simulink model "ROV_Simulation_openloop_ver3_1"  (R2023a)
settings: Solver=ode45  StartTime=0.0  StopTime=Sim.ts  FixedStep=0.01  MaxStep=0.001  MinStep=0.00001  RelTol=1e-3
undefined symbols (not defined in the file): ext, hyd, ics, P0, P1, P10, P2, P3, P4, P5, P6, P7, P8, P9, phy, rb, thrust, VC
libraries: simulink_extras x3, simulink x1
(part 1 of 2)
settings Model: Creator=dmmavani  LastModifiedBy=dmmavani
settings SolverCC: ConcurrentTasks=on  PositivePriorityOrder=on  AutoInsertRateTranBlk=on
settings DataIOCC: InspectSignalLogs=on
settings OptimizationCC: BlockReduction=off  DefaultParameterBehavior=Inlined  EnhancedBackFolding=on  PassReuseOutputArgsAs=Individual arguments  ZeroExternalMemoryAtStartup=off  ZeroInternalMemoryAtStartup=off  OptimizeBlockOrder=speed  DifferentSizesBufferReuse=on  OptimizationCustomize=off  EfficientTunableParamExpr=on
settings DebuggingCC: TasksWithSamePriorityMsg=none  ParameterTunabilityLossMsg=error
settings HardwareCC: ProdBitPerLong=64  ProdLongLongMode=on  ProdHWDeviceType=Intel->x86-64 (Linux 64)
settings SFSimCC: MATLABDynamicMemAlloc=off
settings RTWCC: Description=Embedded Coder  SystemTargetFile=ert.tlc  GenCodeOnly=on  TemplateMakefile=ert_default_tmf  Toolchain=Simulink Real-Time Toolchain  BuildConfiguration=Faster Runs  CodeExecutionProfiling=on  TargetLang=C++
settings CodeAppCC: ForceParamTrailComments=on  IgnoreCustomStorageClasses=off  OperatorAnnotations=on  SimulinkDataObjDesc=on  SFDataObjDesc=on  InsertBlockDesc=on
settings ERTTargetCC: TargetLangStandard=C++03 (ISO)  GenerateSampleERTMain=on  CodeInterfacePackaging=C++ class  InlinedParameterPlacement=NonHierarchical  RootIOFormat=Structure reference  ERTCustomFileTemplate=example_file_process.tlc

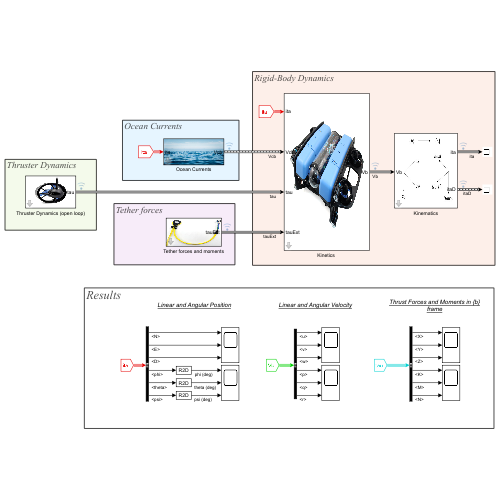
[thumbnail: Simulink's stored preview of the top-level diagram]
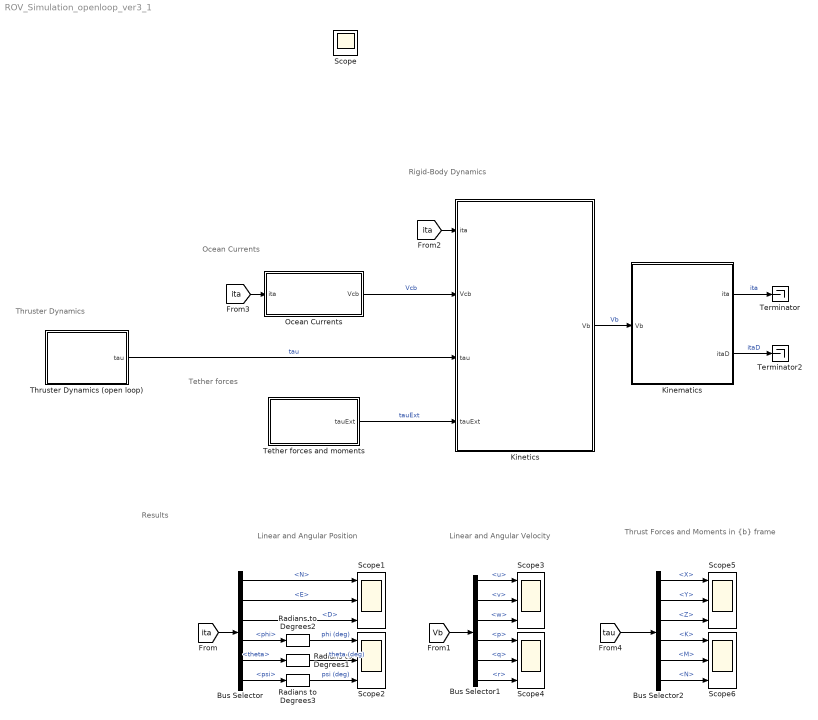
== system ROV_Simulation_openloop_ver3_1 ==
  note: Results
  note: Linear and Angular Position
  note: Tether forces
  note: Thruster Dynamics
  note: Ocean Currents
  note: Rigid-Body Dynamics
  note: Linear and Angular Velocity
  note: Thrust Forces and Moments in {b} frame
  Bus Selector : BusSelector  OutputSignals=N,E,D,phi,theta,psi
  Bus Selector1 : BusSelector  OutputSignals=u,v,w,p,q,r
  Bus Selector2 : BusSelector  OutputSignals=X,Y,Z,K,M,N
  Kinematics : Subsystem  mask{Parameter7=|, North=ics.ita.N, East=ics.ita.E, Down=ics.ita.D, Roll=ics.ita.phi, Pitch=ics.ita.theta, InitialCondition=ics.ita.psi}
      mask Parameter7=|
      | Kinematics block is used to transform velocities from BODY to
      | NED frame.
      |
      | itaD = J(euler) * Vb    ( Velocities in NED frame)
      | J(euler) = Transformation Matrix (function of euler angles)
      | Vb = Velocities in BODY frame.
      mask prompts: North "N :"; East "E :"; Down "D :"; Roll "Roll :"; Pitch "Pitch :"; InitialCondition "Yaw :"
      mask TypeOptions North: Integrator/InitialCondition
      mask TypeOptions East: Integrator1/InitialCondition
      mask TypeOptions Down: Integrator3/InitialCondition
      mask TypeOptions Roll: Integrator4/InitialCondition
      mask TypeOptions Pitch: Integrator5/InitialCondition
      mask TypeOptions InitialCondition: Integrator6/InitialCondition
      mask DialogControl Container4 Prompt: Description
      mask DialogControl Container1 Prompt: Initial Conditions for position and orientation in NED frame
      mask DialogControl Container2 Prompt: Position (meters)
      mask DialogControl Container3 Prompt: Orientation (rad)
      mask Display:
      | image('C:\Users\Dizzy\Documents\Research\MATLAB files\ROV_Simulation\documents\frame_transform_1.png.jpg');
      | port_label('input', 1, 'Vb');
      | port_label('output', 1, 'ita');
      | port_label('output', 2, 'itaD');
  "Kinetics " : Subsystem  mask{Parameter7=|, u_b=ics.vb.u, v_b=ics.vb.v, w_b=ics.vb.w, p_b=ics.vb.p, q_b=ics.vb.q, r_b=ics.vb.r}
      mask Parameter7=|
      | Kinetics block is used to solve the 6DOF equations of motion
      | of a ROV in BODY frame.
      | Block outputs V_b (Velocities in BODY frame).
      mask prompts: u_b "u :"; v_b "v :"; w_b "w :"; p_b "p :"; q_b "q :"; r_b "r :"
      mask TypeOptions u_b: Integrator/InitialCondition
      mask TypeOptions v_b: Integrator1/InitialCondition
      mask TypeOptions w_b: Integrator2/InitialCondition
      mask TypeOptions p_b: Integrator3/InitialCondition
      mask TypeOptions q_b: Integrator4/InitialCondition
      mask TypeOptions r_b: Integrator5/InitialCondition
      mask DialogControl Container4 Prompt: Description
      mask DialogControl InitialCondition Prompt: Initial conditions for velocity of body in {b} frame
      mask DialogControl Container2 Prompt: Linear Velocity  (m/s)
      mask DialogControl Container3 Prompt: Angular Velocity (rad/s)
      mask Display:
      | image('C:\Users\Dizzy\Documents\Research\MATLAB files\ROV_Simulation\documents\heavy-tutorial-21.jpg');
      | port_label('input', 1, 'ita');
      | port_label('input', 2, 'Vcb');
      | port_label('input', 3, 'tau');
      | port_label('input', 4, 'tauExt');
      | port_label('output', 1, 'Vb');
  Ocean Currents : Subsystem  mask{Parameter1=|, Value=VC}
      mask Parameter1=|
      | If the value is equal to 1 then ocean currents is ON.
      | if the value is equal to 0 then ocean currents is OFF.
      mask prompts: Value "Ocean currents (On/Off):"
      mask TypeOptions Value: Constant1/Value
      mask DialogControl Container2 Prompt: Description
      mask Display:
      | image('C:\Users\Dizzy\Documents\Research\MATLAB files\ROV_Simulation\documents\ROV_Simulation_openloop\Images\ocean_currents.jpg');
      | port_label('input', 1, 'ita');
      | port_label('output', 1, 'Vcb');
  Radians to Degrees1 : simulink_extras/Transformations/Radians to Degrees
  Radians to Degrees2 : simulink_extras/Transformations/Radians to Degrees
  Radians to Degrees3 : simulink_extras/Transformations/Radians to Degrees
  Scope{1..6} (6 alike) : Scope  NumInputPorts=3
  Terminator : Terminator
  Terminator2 : Terminator
  Tether forces and moments : Subsystem  mask(Tether forces (external forces)){}
      mask Help:
      | This block is used to compute tether forces acting on ROV in BODY or {b} frame.
      | tauExt = {Xe,Ye,Ze,Ke,Me,Ne}
      | 
      | Tether is modelled using lumped mass approach and there are certain steps to follow to alter the number of nodes for lumped mass tether model.
      | The steps are as follows:
      |     Step 1: Go inside the mask. (click on the bottom left arrow to go inside the mask)
      |     Step 2: Go inside the "tether forces" subsystem block.
      |     Step 3: Go inside the "enable" subsytem variant block.
      |     Step 4: Open MATLAB function block "Tether dynamics" and edit
      |                  the value of "n" for number of nodes.
      | 
      | ** Note **
      | The value of "n" should be two less than the total number of nodes, and must be altered everytime you change its value in workspace. Consequently, it can lead to size missmatch error if not changed.
      mask DialogControl DescGroupVar Prompt: Description
      mask DialogControl Control1 Prompt: Click on help to understand the usage of this block
      mask Display:
      | image('C:\Users\Dizzy\Documents\Research\MATLAB files\ROV_Simulation\documents\ROV_Simulation_openloop\Images\tether.jpg');
      | port_label('output', 1, 'tauExt');
  Thruster Dynamics (open loop) : Subsystem  mask{Parameter2=|, Value=1}
      mask Parameter2=|
      | Pulse input    (Input type = 1)
      | Impulse input (Input type = 0)
      mask prompts: Value "Input type:"
      mask TypeOptions Value: Constant/Value
      mask DialogControl DescGroupVar Prompt: Description
      mask Display:
      | image('C:\Users\Dizzy\Documents\Research\MATLAB files\ROV_Simulation\documents\ROV_Simulation_openloop\Images\T200-Marine-thruster.jpeg');
      | port_label('output', 1, 'tau');
  Scope : Scope
  wires:
  Ocean Currents/1(Vcb) -> "Kinetics "/2(Vcb)  "Vcb"
  [ita] -> Bus Selector/1
  Bus Selector/1 -> Scope1/1  "<N>"
  Bus Selector/2 -> Scope1/2  "<E>"
  Bus Selector/3 -> Scope1/3  "<D>"
  Bus Selector/4 -> Radians to Degrees2/1  "<phi>"
  Radians to Degrees2/1 -> Scope2/1  "phi (deg)"
  Bus Selector/5 -> Radians to Degrees1/1  "<theta>"
  Bus Selector/6 -> Radians to Degrees3/1  "<psi>"
  [Vb] -> Bus Selector1/1
  Bus Selector1/1 -> Scope3/1  "<u>"
  Bus Selector1/2 -> Scope3/2  "<v>"
  Bus Selector1/3 -> Scope3/3  "<w>"
  Bus Selector1/4 -> Scope4/1  "<p>"
  Bus Selector1/5 -> Scope4/2  "<q>"
  Bus Selector1/6 -> Scope4/3  "<r>"
  Kinematics/1(ita) -> Terminator/1  "ita"
  [ita] -> Ocean Currents/1(ita)
  Thruster Dynamics (open loop)/1(tau) -> "Kinetics "/3(tau)  "tau"
  "Kinetics "/1(Vb) -> Kinematics/1(Vb)  "Vb"
  Kinematics/2(itaD) -> Terminator2/1  "itaD"
  [ita] -> "Kinetics "/1(ita)
  [tau] -> Bus Selector2/1
  Bus Selector2/1 -> Scope5/1  "<X>"
  Bus Selector2/2 -> Scope5/2  "<Y>"
  Bus Selector2/3 -> Scope5/3  "<Z>"
  Bus Selector2/4 -> Scope6/1  "<K>"
  Bus Selector2/5 -> Scope6/2  "<M>"
  Bus Selector2/6 -> Scope6/3  "<N>"
  Radians to Degrees1/1 -> Scope2/2  "theta (deg)"
  Radians to Degrees3/1 -> Scope2/3  "psi (deg)"
  Tether forces and moments/1(tauExt) -> "Kinetics "/4(tauExt)  "tauExt"

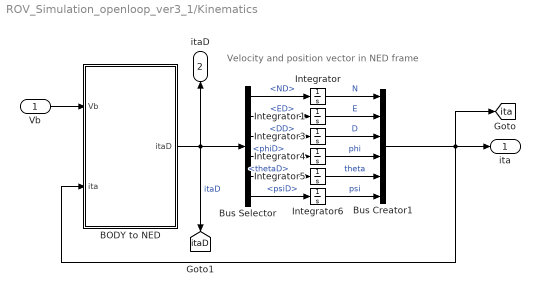
== system ROV_Simulation_openloop_ver3_1/Kinematics ==
  note: Velocity and position vector in
      |  NED frame
  Vb : Inport  OutDataTypeStr=Bus: Vb
  " BODY to NED" : MATLAB Function  TreatAsAtomicUnit=on
  Bus Creator1 : BusCreator  Inputs=6  OutDataTypeStr=Bus: ita
  Bus Selector : BusSelector  OutputSignals=ND,ED,DD,phiD,thetaD,psiD
  Integrator : Integrator  InitialCondition=North  LowerSaturationLimit=ics.N
  Integrator1 : Integrator  InitialCondition=East  LowerSaturationLimit=ics.E
  Integrator3 : Integrator  InitialCondition=Down  LowerSaturationLimit=ics.D
  Integrator4 : Integrator  InitialCondition=Roll  LowerSaturationLimit=ics.phi
  Integrator5 : Integrator  InitialCondition=Pitch  LowerSaturationLimit=ics.theta
  Integrator6 : Integrator  InitialCondition=InitialCondition  LowerSaturationLimit=ics.psi
  ita : Outport  OutDataTypeStr=Bus: ita
  itaD : Outport  Port=2  OutDataTypeStr=Bus: itaD
  tag scope: ita=global, itaD=global
  wires:
  " BODY to NED"/1(itaD) -> Bus Selector/1, [itaD], itaD/1  "itaD"
  Bus Creator1/1 -> [ita], ita/1, " BODY to NED"/2(ita)
  Bus Selector/1 -> Integrator/1  "<ND>"
  Bus Selector/2 -> Integrator1/1  "<ED>"
  Bus Selector/6 -> Integrator6/1  "<psiD>"
  Bus Selector/5 -> Integrator5/1  "<thetaD>"
  Bus Selector/3 -> Integrator3/1  "<DD>"
  Bus Selector/4 -> Integrator4/1  "<phiD>"
  Integrator/1 -> Bus Creator1/1  "N"
  Integrator1/1 -> Bus Creator1/2  "E"
  Integrator3/1 -> Bus Creator1/3  "D"
  Integrator4/1 -> Bus Creator1/4  "phi"
  Integrator5/1 -> Bus Creator1/5  "theta"
  Integrator6/1 -> Bus Creator1/6  "psi"
  Vb/1 -> " BODY to NED"/1(Vb)

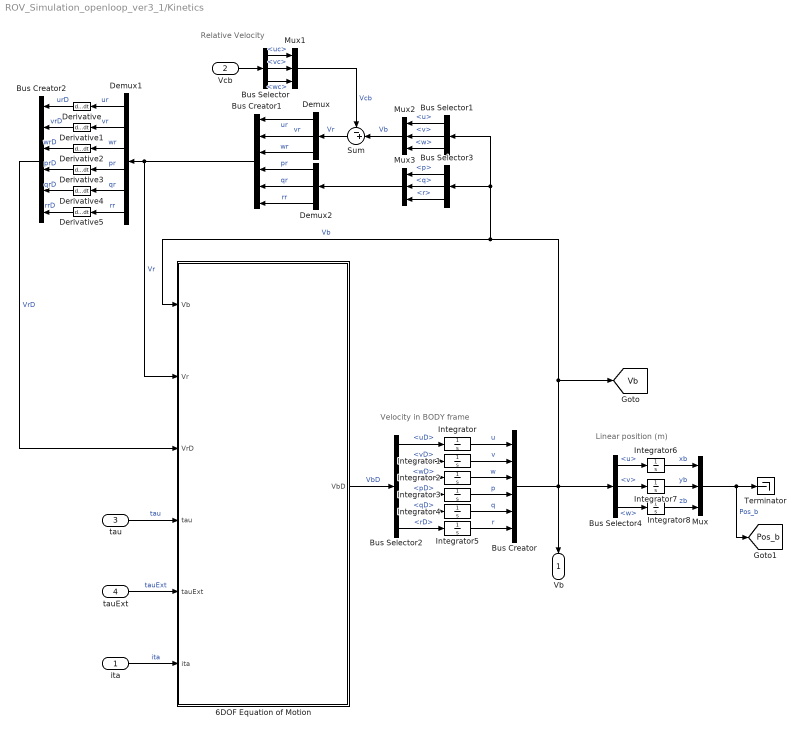
== system ROV_Simulation_openloop_ver3_1/Kinetics  ==
  note: Linear position (m)
  note: Velocity in BODY frame
  note: Relative Velocity
  ita : Inport  OutDataTypeStr=Bus: ita
  Vcb : Inport  Port=2  OutDataTypeStr=Bus: Vcb
  tau : Inport  Port=3  OutDataTypeStr=Bus: tau
  tauExt : Inport  Port=4  OutDataTypeStr=Bus: tauExt
  "6DOF Equation of Motion " : MATLAB Function  TreatAsAtomicUnit=on
  Bus Creator : BusCreator  Inputs=6  OutDataTypeStr=Bus: Vb
  Bus Creator1 : BusCreator  Inputs=6  OutDataTypeStr=Bus: Vr
  Bus Creator2 : BusCreator  Inputs=6  OutDataTypeStr=Bus: VrD
  Bus Selector : BusSelector  OutputSignals=uc,vc,wc
  Bus Selector1 : BusSelector  OutputSignals=u,v,w
  Bus Selector2 : BusSelector  OutputSignals=uD,vD,wD,pD,qD,rD
  Bus Selector3 : BusSelector  OutputSignals=p,q,r
  Bus Selector4 : BusSelector  OutputSignals=u,v,w
  Demux : Demux  Outputs=3
  Demux1 : Demux  Outputs=6
  Demux2 : Demux  Outputs=3
  Derivative{,1..5} (6 alike) : Derivative
  Integrator : Integrator  InitialCondition=u_b  UpperSaturationLimit=ics.sat.umax  LowerSaturationLimit=0
  Integrator1 : Integrator  InitialCondition=v_b  UpperSaturationLimit=ics.sat.vmax  LowerSaturationLimit=0
  Integrator2 : Integrator  InitialCondition=w_b  UpperSaturationLimit=ics.sat.wmax  LowerSaturationLimit=0
  Integrator3 : Integrator  InitialCondition=p_b  UpperSaturationLimit=ics.sat.pmax  LowerSaturationLimit=0
  Integrator4 : Integrator  InitialCondition=q_b  UpperSaturationLimit=ics.sat.qmax  LowerSaturationLimit=0
  Integrator5 : Integrator  InitialCondition=r_b  UpperSaturationLimit=ics.sat.rmax  LowerSaturationLimit=0
  Integrator6 : Integrator  LowerSaturationLimit=0
  Integrator7 : Integrator  LowerSaturationLimit=0
  Integrator8 : Integrator  LowerSaturationLimit=0
  Mux{,1..3} (4 alike) : Mux  Inputs=3
  Sum : Sum  Inputs=-+|
  Terminator : Terminator
  Vb : Outport  OutDataTypeStr=Bus: Vb
  tag scope: Pos_b=global, Vb=global
  wires:
  Mux1/1 -> Sum/1  "Vcb"
  Bus Selector1/1 -> Mux2/1  "<u>"
  Bus Selector1/2 -> Mux2/2  "<v>"
  Bus Selector1/3 -> Mux2/3  "<w>"
  Mux2/1 -> Sum/2  "Vb"
  Bus Creator/1 -> Bus Selector1/1, Bus Selector3/1, "6DOF Equation of Motion "/1(Vb), [Vb], Vb/1, Bus Selector4/1  "Vb"
  ita/1 -> "6DOF Equation of Motion "/6(ita)  "ita"
  tau/1 -> "6DOF Equation of Motion "/4(tau)  "tau"
  "6DOF Equation of Motion "/1(VbD) -> Bus Selector2/1  "VbD"
  Bus Selector2/1 -> Integrator/1  "<uD>"
  Bus Selector2/2 -> Integrator1/1  "<vD>"
  Bus Selector2/3 -> Integrator2/1  "<wD>"
  Bus Selector2/4 -> Integrator3/1  "<pD>"
  Bus Selector2/5 -> Integrator4/1  "<qD>"
  Bus Selector2/6 -> Integrator5/1  "<rD>"
  Vcb/1 -> Bus Selector/1
  Bus Selector/1 -> Mux1/1  "<uc>"
  Bus Selector/2 -> Mux1/2  "<vc>"
  Bus Selector/3 -> Mux1/3  "<wc>"
  Sum/1 -> Demux/1  "Vr"
  Demux/1 -> Bus Creator1/1  "ur"
  Demux/3 -> Bus Creator1/3  "wr"
  Mux3/1 -> Demux2/1
  Demux/2 -> Bus Creator1/2  "vr"
  Demux2/1 -> Bus Creator1/4  "pr"
  Demux2/2 -> Bus Creator1/5  "qr"
  Demux2/3 -> Bus Creator1/6  "rr"
  Integrator/1 -> Bus Creator/1  "u"
  Integrator1/1 -> Bus Creator/2  "v"
  Integrator2/1 -> Bus Creator/3  "w"
  Integrator3/1 -> Bus Creator/4  "p"
  Integrator4/1 -> Bus Creator/5  "q"
  Integrator5/1 -> Bus Creator/6  "r"
  Bus Selector3/2 -> Mux3/2  "<q>"
  Bus Selector3/3 -> Mux3/3  "<r>"
  Bus Selector3/1 -> Mux3/1  "<p>"
  Bus Selector4/1 -> Integrator6/1  "<u>"
  Bus Selector4/2 -> Integrator7/1  "<v>"
  Bus Selector4/3 -> Integrator8/1  "<w>"
  Integrator6/1 -> Mux/1  "xb"
  Integrator7/1 -> Mux/2  "yb"
  Integrator8/1 -> Mux/3  "zb"
  Mux/1 -> [Pos_b], Terminator/1  "Pos_b"
  Bus Creator1/1 -> Demux1/1, "6DOF Equation of Motion "/2(Vr)  "Vr"
  Demux1/1 -> Derivative/1  "ur"
  Derivative/1 -> Bus Creator2/1  "urD"
  Demux1/2 -> Derivative1/1  "vr"
  Derivative1/1 -> Bus Creator2/2  "vrD"
  Demux1/3 -> Derivative2/1  "wr"
  Derivative2/1 -> Bus Creator2/3  "wrD"
  Demux1/4 -> Derivative3/1  "pr"
  Derivative3/1 -> Bus Creator2/4  "prD"
  Demux1/5 -> Derivative4/1  "qr"
  Derivative4/1 -> Bus Creator2/5  "qrD"
  Demux1/6 -> Derivative5/1  "rr"
  Derivative5/1 -> Bus Creator2/6  "rrD"
  Bus Creator2/1 -> "6DOF Equation of Motion "/3(VrD)  "VrD"
  tauExt/1 -> "6DOF Equation of Motion "/5(tauExt)  "tauExt"

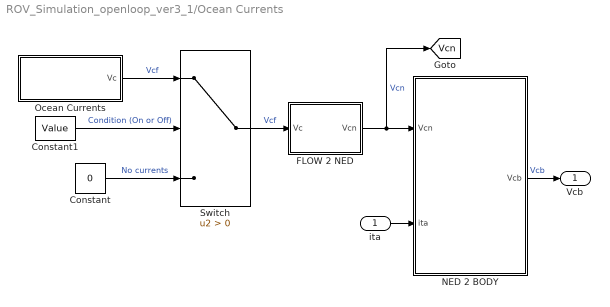
== system ROV_Simulation_openloop_ver3_1/Ocean Currents ==
  ita : Inport  OutDataTypeStr=Bus: ita
  Constant : Constant  Value=0
  Constant1 : Constant  Value=Value
  FLOW 2 NED : MATLAB Function  TreatAsAtomicUnit=on
  NED 2 BODY : MATLAB Function  TreatAsAtomicUnit=on
  Ocean Currents : Subsystem  Variant=on
  Switch : Switch  Criteria=u2 > Threshold  SaturateOnIntegerOverflow=off  InputSameDT=off
  Vcb : Outport  OutDataTypeStr=Bus: Vcb
  tag scope: Vcn=global
  wires:
  Ocean Currents/1(Vc) -> Switch/1  "Vcf"
  Constant/1 -> Switch/3  "No currents"
  Switch/1 -> FLOW 2 NED/1(Vc)  "Vcf"
  Constant1/1 -> Switch/2  "Condition (On or Off)"
  FLOW 2 NED/1(Vcn) -> NED 2 BODY/1(Vcn), [Vcn]  "Vcn"
  ita/1 -> NED 2 BODY/2(ita)
  NED 2 BODY/1(Vcb) -> Vcb/1  "Vcb"

== system ROV_Simulation_openloop_ver3_1/Tether forces and moments ==
  Tether Forces : Subsystem  Variant=on
  tauExt : Outport
  wires:
  Tether Forces/1(tauExt) -> tauExt/1

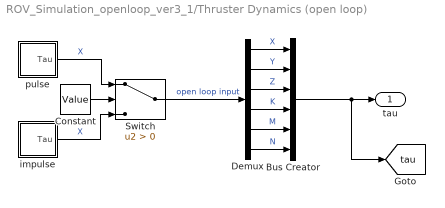
== system ROV_Simulation_openloop_ver3_1/Thruster Dynamics (open loop) ==
  Bus Creator : BusCreator  Inputs=6  OutDataTypeStr=Bus: tau
  Constant : Constant  Value=Value
  Demux : Demux  Outputs=6
  Switch : Switch  Criteria=u2 > Threshold  SaturateOnIntegerOverflow=off  InputSameDT=off
  impulse : Subsystem
  pulse : Subsystem
  tau : Outport  OutDataTypeStr=Bus: tau
  tag scope: tau=global
  wires:
  Demux/2 -> Bus Creator/2  "Y"
  Demux/3 -> Bus Creator/3  "Z"
  Demux/4 -> Bus Creator/4  "K"
  Demux/5 -> Bus Creator/5  "M"
  Demux/6 -> Bus Creator/6  "N"
  Bus Creator/1 -> [tau], tau/1
  Demux/1 -> Bus Creator/1  "X"
  pulse/1(Tau) -> Switch/1  "X"
  impulse/1(Tau) -> Switch/3  "X"
  Constant/1 -> Switch/2
  Switch/1 -> Demux/1  "open loop input"

== system ROV_Simulation_openloop_ver3_1/Ocean Currents/Ocean Currents ==
  VC_CONSTANT : Subsystem  VariantControl=VC_CONSTANT
  VC_RANDOM : Subsystem  VariantControl=VC_RANDOM
  Vc : Outport

== system ROV_Simulation_openloop_ver3_1/Tether forces and moments/Tether Forces ==
  Disable : Subsystem  VariantControl=TETHER_DISABLE
  Enable : Subsystem  VariantControl=TETHER_ENABLE
  tauExt : Outport

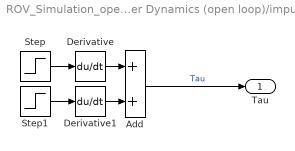
== system ROV_Simulation_openloop_ver3_1/Thruster Dynamics (open loop)/impulse ==
  Add : Sum
  Derivative : Derivative
  Derivative1 : Derivative
  Step : Step  Time=thrust.start  Before=-thrust.control.Tau  After=-thrust.control.Tau+thrust.control.Tau  SampleTime=0
  Step1 : Step  Time=thrust.start + thrust.duration  Before=thrust.control.Tau  After=0  SampleTime=0
  Tau : Outport
  wires:
  Add/1 -> Tau/1  "Tau"
  Step/1 -> Derivative/1
  Derivative/1 -> Add/1
  Step1/1 -> Derivative1/1
  Derivative1/1 -> Add/2

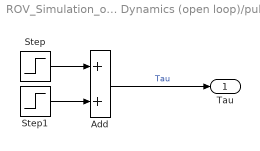
== system ROV_Simulation_openloop_ver3_1/Thruster Dynamics (open loop)/pulse ==
  Add : Sum
  Step : Step  Time=thrust.start  Before=-thrust.control.Tau  After=-thrust.control.Tau+thrust.control.Tau  SampleTime=0
  Step1 : Step  Time=thrust.duration+thrust.start  Before=thrust.control.Tau  After=0  SampleTime=0
  Tau : Outport
  wires:
  Step1/1 -> Add/2
  Step/1 -> Add/1
  Add/1 -> Tau/1  "Tau"

== system ROV_Simulation_openloop_ver3_1/Ocean Currents/Ocean Currents/VC_CONSTANT ==
  Constant : Constant  Value=hyd.ocean.flow.constant
  Vc : Outport
  wires:
  Constant/1 -> Vc/1

== system ROV_Simulation_openloop_ver3_1/Ocean Currents/Ocean Currents/VC_RANDOM ==
  Band-Limited White Noise : simulink/Sources/Band-Limited White Noise  Cov=hyd.ocean.flow.noise.power  Ts=hyd.ocean.flow.noise.ts  seed=[23341]
  Gauss-Markov first order method : TransferFcn  Denominator=[1 hyd.ocean.flow.varying.mu]
  Saturation : Saturate  UpperLimit=hyd.ocean.flow.varying.Vmax  LowerLimit=hyd.ocean.flow.varying.Vmin
  Vc : Outport
  wires:
  Band-Limited White Noise/1 -> Gauss-Markov first order method/1
  Gauss-Markov first order method/1 -> Saturation/1  "Unconstrained currents"
  Saturation/1 -> Vc/1  "Constrained currents"

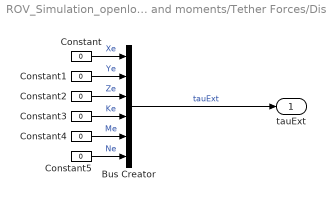
== system ROV_Simulation_openloop_ver3_1/Tether forces and moments/Tether Forces/Disable ==
  Bus Creator : BusCreator  Inputs=6  OutDataTypeStr=Bus: tauExt
  Constant{,1..5} (6 alike) : Constant  Value=0
  tauExt : Outport  OutDataTypeStr=Bus: tauExt
  wires:
  Constant/1 -> Bus Creator/1  "Xe"
  Constant2/1 -> Bus Creator/3  "Ze"
  Constant3/1 -> Bus Creator/4  "Ke"
  Bus Creator/1 -> tauExt/1  "tauExt"
  Constant1/1 -> Bus Creator/2  "Ye"
  Constant4/1 -> Bus Creator/5  "Me"
  Constant5/1 -> Bus Creator/6  "Ne"

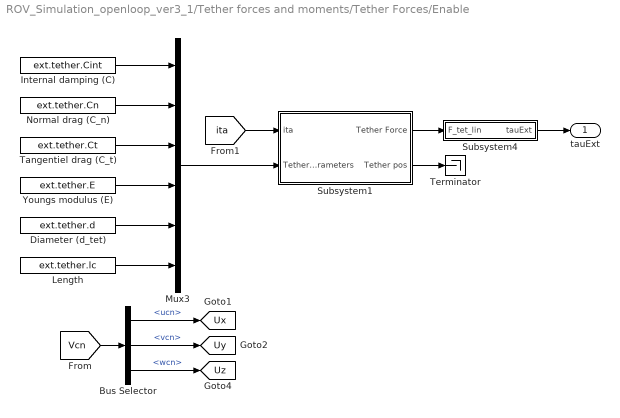
== system ROV_Simulation_openloop_ver3_1/Tether forces and moments/Tether Forces/Enable ==
  Bus Selector : BusSelector  OutputSignals=ucn,vcn,wcn
  Diameter (d_tet) : Constant  Value=ext.tether.d
  Internal damping (C) : Constant  Value=ext.tether.Cint
  Length : Constant  Value=ext.tether.lc
  Mux3 : Mux  Inputs=6
  Normal drag (C_n) : Constant  Value=ext.tether.Cn
  Subsystem1 : Subsystem
  Subsystem4 : Subsystem
  Tangentiel drag (C_t) : Constant  Value=ext.tether.Ct
  Terminator : Terminator
  Youngs modulus (E) : Constant  Value=ext.tether.E
  tauExt : Outport  OutDataTypeStr=Bus: tauExt
  tag scope: Ux=global, Uy=global, Uz=global
  wires:
  Youngs modulus (E)/1 -> Mux3/4
  Mux3/1 -> Subsystem1/2(Tether_Parameters)
  Internal damping (C)/1 -> Mux3/1
  Subsystem1/2(Tether pos) -> Terminator/1
  Diameter (d_tet)/1 -> Mux3/5
  Tangentiel drag (C_t)/1 -> Mux3/3
  Length/1 -> Mux3/6
  Normal drag (C_n)/1 -> Mux3/2
  Subsystem4/1(tauExt) -> tauExt/1
  Subsystem1/1(Tether Force) -> Subsystem4/1(F_tet_lin)
  [Vcn] -> Bus Selector/1
  Bus Selector/1 -> [Ux]  "<ucn>"
  Bus Selector/2 -> [Uy]  "<vcn>"
  Bus Selector/3 -> [Uz]  "<wcn>"
  [ita] -> Subsystem1/1(ita)

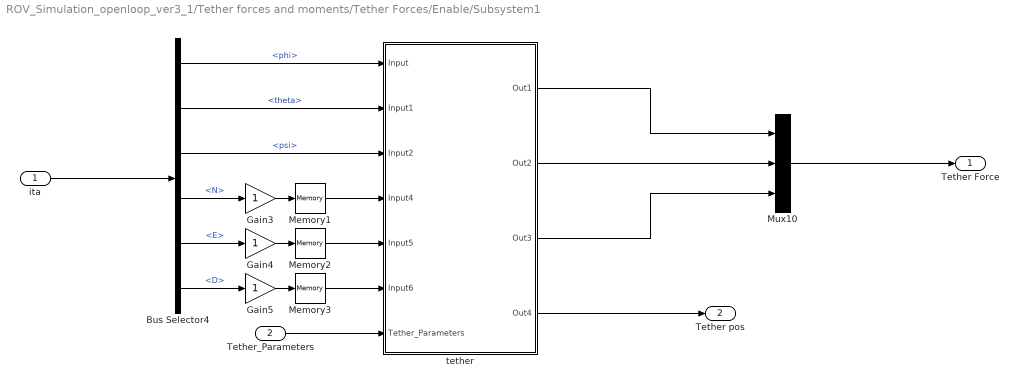
== system ROV_Simulation_openloop_ver3_1/Tether forces and moments/Tether Forces/Enable/Subsystem1 ==
  ita : Inport  OutDataTypeStr=Bus: ita
  Tether_Parameters : Inport  Port=2
  Bus Selector4 : BusSelector  OutputSignals=phi,theta,psi,N,E,D
  Gain3 : Gain
  Gain4 : Gain
  Gain5 : Gain
  Memory1 : Memory  InitialCondition=P10(1)
  Memory2 : Memory  InitialCondition=P10(2)
  Memory3 : Memory  InitialCondition=P10(3)
  Mux10 : Mux  Inputs=3
  tether : Subsystem
  Tether Force : Outport
  Tether pos : Outport  Port=2
  wires:
  Memory3/1 -> tether/6(Input6)
  Memory2/1 -> tether/5(Input5)
  Memory1/1 -> tether/4(Input4)
  Bus Selector4/1 -> tether/1(Input)  "<phi>"
  Bus Selector4/2 -> tether/2(Input1)  "<theta>"
  Bus Selector4/3 -> tether/3(Input2)  "<psi>"
  Tether_Parameters/1 -> tether/7(Tether_Parameters)
  Gain3/1 -> Memory1/1
  Gain4/1 -> Memory2/1
  Gain5/1 -> Memory3/1
  tether/1(Out1) -> Mux10/1
  tether/2(Out2) -> Mux10/2
  tether/3(Out3) -> Mux10/3
  Mux10/1 -> Tether Force/1
  tether/4(Out4) -> Tether pos/1
  Bus Selector4/4 -> Gain3/1  "<N>"
  Bus Selector4/5 -> Gain4/1  "<E>"
  Bus Selector4/6 -> Gain5/1  "<D>"
  ita/1 -> Bus Selector4/1

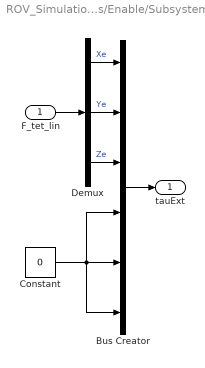
== system ROV_Simulation_openloop_ver3_1/Tether forces and moments/Tether Forces/Enable/Subsystem4 ==
  F_tet_lin : Inport
  Bus Creator : BusCreator  Inputs=6  OutDataTypeStr=Bus: tauExt
      settings: InheritFromInputs=off
  Constant : Constant  Value=0
  Demux : Demux  Outputs=3
  tauExt : Outport  OutDataTypeStr=Bus: tauExt
  wires:
  Constant/1 -> Bus Creator/6, Bus Creator/4, Bus Creator/5
  Bus Creator/1 -> tauExt/1
  Demux/1 -> Bus Creator/1  "Xe"
  Demux/2 -> Bus Creator/2  "Ye"
  Demux/3 -> Bus Creator/3  "Ze"
  F_tet_lin/1 -> Demux/1

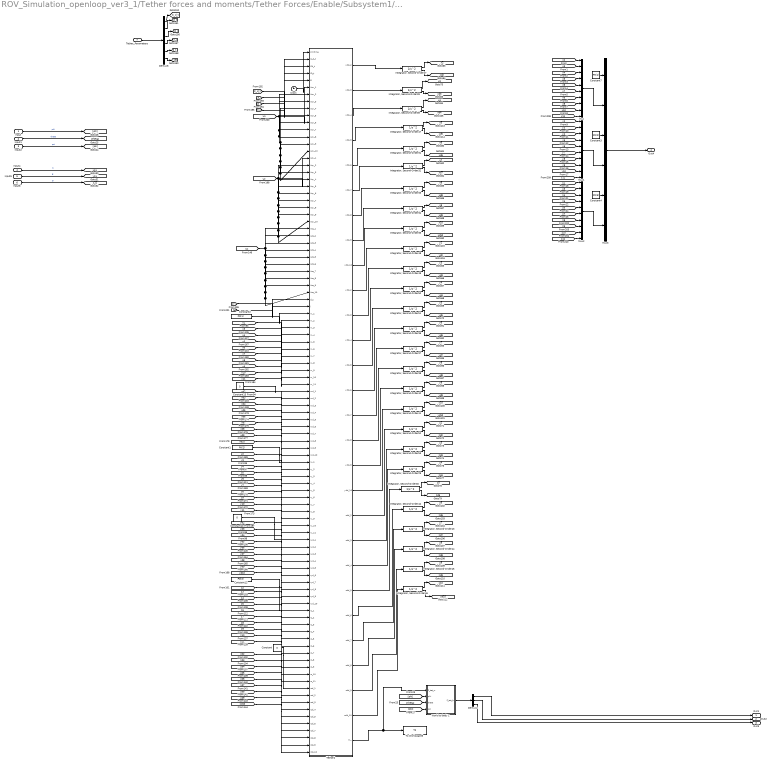
== system ROV_Simulation_openloop_ver3_1/Tether forces and moments/Tether Forces/Enable/Subsystem1/tether ==
  Input : Inport
  Input1 : Inport  Port=2
  Input2 : Inport  Port=3
  Input4 : Inport  Port=4
  Input5 : Inport  Port=5
  Input6 : Inport  Port=6
  Tether_Parameters : Inport  Port=7
  Clock : Clock
  Constant : Constant  Value=0
  Constant1 : Constant  Value=P0(2)
  Constant10 : Constant  Value=0
  Constant12 : Constant  Value=P0(3)
  Constant13 : Constant  Value=0
  Constant2 : Constant  Value=P0(1)
  Constant3 : Constant  Value=P0(2)
  Constant4 : Constant  Value=P0(3)
  Constant7 : Constant  Value=P0(1)
  Demux4 : Demux  Outputs=3
  Demux6 : Demux  Outputs=6
  "Integrator, Second-Order27" : SecondOrderIntegrator  ICX=P1(1)
  "Integrator, Second-Order28" : SecondOrderIntegrator  ICX=P2(1)
  "Integrator, Second-Order29" : SecondOrderIntegrator  ICX=P3(3)
  "Integrator, Second-Order30" : SecondOrderIntegrator  ICX=P4(3)
  "Integrator, Second-Order31" : SecondOrderIntegrator  ICX=P5(1)
  "Integrator, Second-Order32" : SecondOrderIntegrator  ICX=P6(1)
  "Integrator, Second-Order33" : SecondOrderIntegrator  ICX=P7(1)
  "Integrator, Second-Order34" : SecondOrderIntegrator  ICX=P8(1)  UpperLimitX=100  LowerLimitX=-100  UpperLimitDXDT=10  LowerLimitDXDT=-10
  "Integrator, Second-Order35" : SecondOrderIntegrator  ICX=P9(1)
  "Integrator, Second-Order36" : SecondOrderIntegrator  ICX=P5(2)
  "Integrator, Second-Order37" : SecondOrderIntegrator  ICX=P6(2)
  "Integrator, Second-Order38" : SecondOrderIntegrator  ICX=P7(2)
  "Integrator, Second-Order39" : SecondOrderIntegrator  ICX=P3(1)
  "Integrator, Second-Order40" : SecondOrderIntegrator  ICX=P8(2)
  "Integrator, Second-Order41" : SecondOrderIntegrator  ICX=P9(2)
  "Integrator, Second-Order42" : SecondOrderIntegrator  ICX=P5(3)
  "Integrator, Second-Order43" : SecondOrderIntegrator  ICX=P6(3)
  "Integrator, Second-Order44" : SecondOrderIntegrator  ICX=P7(3)
  "Integrator, Second-Order45" : SecondOrderIntegrator  ICX=P8(3)
  "Integrator, Second-Order46" : SecondOrderIntegrator  ICX=P9(3)
  "Integrator, Second-Order47" : SecondOrderIntegrator  ICX=P4(1)
  "Integrator, Second-Order48" : SecondOrderIntegrator  ICX=P1(2)
  "Integrator, Second-Order49" : SecondOrderIntegrator  ICX=P2(2)
  "Integrator, Second-Order50" : SecondOrderIntegrator  ICX=P3(2)
  "Integrator, Second-Order51" : SecondOrderIntegrator  ICX=P4(2)
  "Integrator, Second-Order52" : SecondOrderIntegrator  ICX=P1(3)
  "Integrator, Second-Order53" : SecondOrderIntegrator  ICX=P2(3)
  Mux : Mux  Inputs=10
  Mux1 : Mux  Inputs=10
  Mux2 : Mux  Inputs=10
  Mux3 : Mux  Inputs=6
  Tether2 : MATLAB Function  TreatAsAtomicUnit=on
  To Workspace3 : ToWorkspace  VariableName=T2  SaveFormat=Timeseries  SampleTime=-1
  World to body 1 : MATLAB Function  TreatAsAtomicUnit=on
  Out1 : Outport
  Out2 : Outport  Port=2
  Out3 : Outport  Port=3
  Out4 : Outport  Port=4
  tag scope: C_d_t=global, Cd_t=global, Ct_t=global, Em_t=global, I_tet=global, d_t=global, x10=global, x11=global, x2=global, x3=global, x4=global, x5=global, x6=global, x7=global, x8=global, x9=global, xd10=global, xd2=global, xd3=global, xd4=global, xd5=global, xd6=global, xd7=global, xd8=global, xd9=global, y10=global, y11=global, y2=global, y3=global, y4=global, y5=global, y6=global, y7=global, y8=global, y9=global, yd10=global, yd2=global, yd3=global, yd4=global, yd5=global, yd6=global, yd7=global, yd8=global, yd9=global, z10=global, z11=global, z2=global, z3=global, z4=global, z5=global, z6=global, z7=global, z8=global, z9=global, zd10=global, zd2=global, zd3=global, zd4=global, zd5=global, zd6=global, zd7=global, zd8=global, zd9=global
  wires:
  Input/1 -> [phi]  "phi"
  Input1/1 -> [theta]  "theta"
  Input2/1 -> [psi]  "psi"
  Input4/1 -> [x11]  "N"
  Input5/1 -> [y11]  "E"
  Input6/1 -> [z11]  "D"
  "Integrator, Second-Order46"/1 -> [z10]
  "Integrator, Second-Order52"/1 -> [z2]
  [zd7] -> Tether2/97(rzd_7)
  "Integrator, Second-Order28"/2 -> [xd3]
  "Integrator, Second-Order36"/1 -> [y6]
  "Integrator, Second-Order32"/1 -> [x7]
  [yd7] -> Tether2/76(ryd_7)
  [zd3] -> Tether2/93(rzd_3)
  Constant12/1 -> Tether2/80(rz_1)
  "Integrator, Second-Order29"/2 -> [zd4]
  "Integrator, Second-Order29"/1 -> [z4]
  "Integrator, Second-Order35"/2 -> [xd10]
  [y5] -> Tether2/63(ry_5)
  "Integrator, Second-Order52"/2 -> [zd2]
  [z8] -> Tether2/87(rz_8)
  "Integrator, Second-Order50"/1 -> [y4]
  [y6] -> Tether2/64(ry_6)
  [xd5] -> Tether2/53(rxd_5)
  "Integrator, Second-Order50"/2 -> [yd4]
  "Integrator, Second-Order53"/1 -> [z3]
  [zd5] -> Tether2/95(rzd_5)
  [zd10] -> Tether2/100(rzd_10)
  [xd9] -> Tether2/57(rxd_9)
  [zd6] -> Tether2/96(rzd_6)
  [yd3] -> Tether2/72(ryd_3)
  "Integrator, Second-Order41"/2 -> [yd10]
  [z9] -> Tether2/88(rz_9)
  "Integrator, Second-Order38"/1 -> [y8]
  "Integrator, Second-Order31"/2 -> [xd6]
  "Integrator, Second-Order33"/2 -> [xd8]
  [yd8] -> Tether2/77(ryd_8)
  "Integrator, Second-Order41"/1 -> [y10]
  "Integrator, Second-Order30"/1 -> [z5]
  Constant1/1 -> Tether2/59(ry_1)
  [y9] -> Tether2/67(ry_9)
  "Integrator, Second-Order46"/2 -> [zd10]
  [yd10] -> Tether2/79(ryd_10)
  [z4] -> Tether2/83(rz_4)
  [y10] -> Tether2/68(ry_10)
  "Integrator, Second-Order48"/1 -> [y2]
  "Integrator, Second-Order45"/2 -> [zd9]
  [zd4] -> Tether2/94(rzd_4)
  [z11] -> Tether2/90(rz_11)
  "Integrator, Second-Order47"/2 -> [xd5]
  [y4] -> Tether2/62(ry_4)
  "Integrator, Second-Order31"/1 -> [x6]
  [z3] -> Tether2/82(rz_3)
  [xd4] -> Tether2/52(rxd_4)
  "Integrator, Second-Order37"/2 -> [yd7]
  [x7] -> Tether2/44(rx_7)
  [zd9] -> Tether2/99(rzd_9)
  [x3] -> Tether2/40(rx_3)
  [yd5] -> Tether2/74(ryd_5)
  "Integrator, Second-Order44"/2 -> [zd8]
  "Integrator, Second-Order40"/1 -> [y9]
  "Integrator, Second-Order27"/1 -> [x2]
  "Integrator, Second-Order48"/2 -> [yd2]
  [yd2] -> Tether2/71(ryd_2)
  "Integrator, Second-Order51"/2 -> [yd5]
  "Integrator, Second-Order36"/2 -> [yd6]
  "Integrator, Second-Order47"/1 -> [x5]
  "Integrator, Second-Order49"/1 -> [y3]
  "Integrator, Second-Order32"/2 -> [xd7]
  [x4] -> Tether2/41(rx_4)
  "Integrator, Second-Order45"/1 -> [z9]
  [xd8] -> Tether2/56(rxd_8)
  "Integrator, Second-Order37"/1 -> [y7]
  [z6] -> Tether2/85(rz_6)
  "Integrator, Second-Order40"/2 -> [yd9]
  "Integrator, Second-Order43"/1 -> [z7]
  "Integrator, Second-Order51"/1 -> [y5]
  Constant2/1 -> Tether2/38(rx_1)
  "Integrator, Second-Order34"/1 -> [x9]
  "Integrator, Second-Order44"/1 -> [z8]
  "Integrator, Second-Order28"/1 -> [x3]
  [z5] -> Tether2/84(rz_5)
  "Integrator, Second-Order39"/1 -> [x4]
  [z7] -> Tether2/86(rz_7)
  [z2] -> Tether2/81(rz_2)
  [xd6] -> Tether2/54(rxd_6)
  "Integrator, Second-Order34"/2 -> [xd9]
  [yd4] -> Tether2/73(ryd_4)
  [x6] -> Tether2/43(rx_6)
  [zd8] -> Tether2/98(rzd_8)
  [x8] -> Tether2/45(rx_8)
  [xd10] -> Tether2/58(rxd_10)
  [x5] -> Tether2/42(rx_5)
  [y7] -> Tether2/65(ry_7)
  [yd6] -> Tether2/75(ryd_6)
  [zd2] -> Tether2/92(rzd_2)
  "Integrator, Second-Order35"/1 -> [x10]
  [xd3] -> Tether2/51(rxd_3)
  "Integrator, Second-Order30"/2 -> [zd5]
  [y2] -> Tether2/60(ry_2)
  "Integrator, Second-Order49"/2 -> [yd3]
  "Integrator, Second-Order27"/2 -> [xd2]
  [y11] -> Tether2/69(ry_11)
  [xd7] -> Tether2/55(rxd_7)
  [yd9] -> Tether2/78(ryd_9)
  [y8] -> Tether2/66(ry_8)
  [z10] -> Tether2/89(rz_10)
  "Integrator, Second-Order42"/2 -> [zd6]
  [x10] -> Tether2/47(rx_10)
  [x2] -> Tether2/39(rx_2)
  [Uz] -> Tether2/35(Ucz_10), Tether2/34(Ucz_9), Tether2/33(Ucz_8), Tether2/32(Ucz_7), Tether2/31(Ucz_6), Tether2/30(Ucz_5), Tether2/29(Ucz_4), Tether2/28(Ucz_3), Tether2/27(Ucz_2), Tether2/26(Ucz_1)
  [x11] -> Tether2/48(rx_11)
  "Integrator, Second-Order33"/1 -> [x8]
  "Integrator, Second-Order39"/2 -> [xd4]
  "Integrator, Second-Order38"/2 -> [yd8]
  [xd2] -> Tether2/50(rxd_2)
  "Integrator, Second-Order43"/2 -> [zd7]
  "Integrator, Second-Order53"/2 -> [zd3]
  [y3] -> Tether2/61(ry_3)
  "Integrator, Second-Order42"/1 -> [z6]
  [x9] -> Tether2/46(rx_9)
  [Ux] -> Tether2/15(Ucx_10), Tether2/14(Ucx_9), Tether2/13(Ucx_8), Tether2/12(Ucx_7), Tether2/11(Ucx_6), Tether2/10(Ucx_5), Tether2/9(Ucx_4), Tether2/8(Ucx_3), Tether2/7(Ucx_2), Tether2/6(Ucx_1)
  [I_tet] -> Tether2/37(l)
  [psi] -> World to body 1/4(psi)
  World to body 1/1(F_tet_b) -> Demux4/1
  [theta] -> World to body 1/3(theta)
  [phi] -> World to body 1/2(phi)
  Tether2/28(Tix) -> World to body 1/1(F_tet_w), To Workspace3/1
  Demux4/1 -> Out1/1
  Demux4/3 -> Out3/1
  Demux4/2 -> Out2/1
  [Uy] -> Tether2/25(Ucy_10), Tether2/24(Ucy_9), Tether2/23(Ucy_8), Tether2/22(Ucy_7), Tether2/21(Ucy_6), Tether2/20(Ucy_5), Tether2/19(Ucy_4), Tether2/18(Ucy_3), Tether2/17(Ucy_2), Tether2/16(Ucy_1)
  [d_t] -> Tether2/36(d_t)
  [Cd_t] -> Tether2/3(Cd_t)
  [Ct_t] -> Tether2/4(Ct_t)
  [Em_t] -> Tether2/5(E)
  Demux6/6 -> [I_tet]
  Demux6/3 -> [Ct_t]
  Tether_Parameters/1 -> Demux6/1
  Demux6/2 -> [Cd_t]
  Demux6/5 -> [d_t]
  Demux6/4 -> [Em_t]
  [C_d_t] -> Tether2/2(C_d_t)
  Demux6/1 -> [C_d_t]
  Tether2/5(xdd_6) -> "Integrator, Second-Order31"/1
  Tether2/6(xdd_7) -> "Integrator, Second-Order32"/1
  Tether2/7(xdd_8) -> "Integrator, Second-Order33"/1
  Tether2/8(xdd_9) -> "Integrator, Second-Order34"/1
  Tether2/9(xdd_10) -> "Integrator, Second-Order35"/1
  Tether2/10(ydd_2) -> "Integrator, Second-Order48"/1
  Tether2/11(ydd_3) -> "Integrator, Second-Order49"/1
  Tether2/12(ydd_4) -> "Integrator, Second-Order50"/1
  Tether2/13(ydd_5) -> "Integrator, Second-Order51"/1
  Tether2/14(ydd_6) -> "Integrator, Second-Order36"/1
  Tether2/15(ydd_7) -> "Integrator, Second-Order37"/1
  Tether2/16(ydd_8) -> "Integrator, Second-Order38"/1
  Tether2/17(ydd_9) -> "Integrator, Second-Order40"/1
  Tether2/18(ydd_10) -> "Integrator, Second-Order41"/1
  Tether2/19(zdd_2) -> "Integrator, Second-Order52"/1
  Tether2/20(zdd_3) -> "Integrator, Second-Order53"/1
  Tether2/21(zdd_4) -> "Integrator, Second-Order29"/1
  Tether2/22(zdd_5) -> "Integrator, Second-Order30"/1
  Tether2/23(zdd_6) -> "Integrator, Second-Order42"/1
  Tether2/24(zdd_7) -> "Integrator, Second-Order43"/1
  Tether2/25(zdd_8) -> "Integrator, Second-Order44"/1
  Tether2/26(zdd_9) -> "Integrator, Second-Order45"/1
  Tether2/27(zdd_10) -> "Integrator, Second-Order46"/1
  Tether2/1(xdd_2) -> "Integrator, Second-Order27"/1
  Tether2/2(xdd_3) -> "Integrator, Second-Order28"/1
  Tether2/3(xdd_4) -> "Integrator, Second-Order39"/1
  Tether2/4(xdd_5) -> "Integrator, Second-Order47"/1
  Constant/1 -> Tether2/91(rzd_1)
  Constant10/1 -> Tether2/70(ryd_1)
  Constant13/1 -> Tether2/49(rxd_1)
  [x2] -> Mux/1
  [x3] -> Mux/2
  [x4] -> Mux/3
  [x5] -> Mux/4
  [x6] -> Mux/5
  [x7] -> Mux/6
  [x8] -> Mux/7
  [x9] -> Mux/8
  [x10] -> Mux/9
  [y9] -> Mux1/8
  [y5] -> Mux1/4
  [y4] -> Mux1/3
  [y3] -> Mux1/2
  [y8] -> Mux1/7
  [y7] -> Mux1/6
  [y10] -> Mux1/9
  [y6] -> Mux1/5
  [y2] -> Mux1/1
  [z9] -> Mux2/8
  [z5] -> Mux2/4
  [z4] -> Mux2/3
  [z3] -> Mux2/2
  [z8] -> Mux2/7
  [z7] -> Mux2/6
  [z10] -> Mux2/9
  [z6] -> Mux2/5
  [z2] -> Mux2/1
  [x11] -> Mux/10
  [y11] -> Mux1/10
  [z11] -> Mux2/10
  Mux/1 -> Mux3/2
  Mux1/1 -> Mux3/4
  Mux2/1 -> Mux3/6
  Mux3/1 -> Out4/1
  Constant7/1 -> Mux3/1
  Constant3/1 -> Mux3/3
  Constant4/1 -> Mux3/5
  Clock/1 -> Tether2/1(simtime)

== matlab function ROV_Simulation_openloop_ver3_1/Kinematics/ BODY to NED ==
  data: itaD output Bus: itaD size=1; Vb input Bus: Vb size=1; ita input Bus: ita
function itaD = Vn(Vb,ita)

vb = [Vb.u,Vb.v,Vb.w,Vb.p,Vb.q,Vb.r]';

% Euler angles
phi = ita.phi;
theta = ita.theta;
psi = ita.psi;

% Rotational matrices (Linear & angular)
Rbn = rotbn(phi,theta,psi);
Tbn = tbn(phi,theta);

% J is transformation matrix
J = [Rbn,zeros(3);zeros(3),Tbn];

% if t>40
%     a=3;
% end

z = J*vb;       % Transformation of velocity from {b} to {n} frame

% Velocity of ROV in NED / {n} frame 
itaD.ND = z(1);
itaD.ED = z(2);
itaD.DD = z(3);
itaD.phiD = z(4);
itaD.thetaD = z(5);
itaD.psiD = z(6);

== matlab function ROV_Simulation_openloop_ver3_1/Ocean Currents/FLOW 2 NED ==
  data: Vc input; Vcn output Bus: Vcn; hyd parameter
function Vcn = f2e(Vc,hyd)

Rfn = R_alpha(hyd)'*R_beta(hyd)';

xx = Rfn * [Vc,0,0]';        % Velocity vector in {n} frame

% Ocean current in NED / {n} frame
Vcn.ucn = xx(1);
Vcn.vcn = xx(2);
Vcn.wcn = xx(3);

== matlab function ROV_Simulation_openloop_ver3_1/Kinetics /6DOF Equation of Motion  ==
  data: Vb input Bus: Vb size=1; Vr input Bus: Vr size=1; VrD input Bus: VrD; tau input Bus: tau size=1; VbD output Bus: VbD size=1; tauExt input Bus: tauExt; ita input Bus: ita size=1; rb parameter; hyd parameter; phy parameter
function VbD = eomRB(Vb, Vr, VrD, tau, tauExt, ita, rb, hyd, phy)

% Equation of motion or kinetic equation can be derived using Mrb (Mass
% matrix), Crb (Coriolis-Centripetal force) and vb (velocity of vehicle in
% body-fixed frame {b}
% EOM is Mrb*vDot + Crb(vb)*vb = tau_RB       


vb = [Vb.u,Vb.v,Vb.w,Vb.p,Vb.q,Vb.r]';          % velocity in body frame
vr = [Vr.ur,Vr.vr,Vr.wr,Vr.pr,Vr.qr,Vr.rr]';    % relative velocity between ocean currents and ROV
vrd = [VrD.urD, VrD.vrD, VrD.wrD, VrD.prD, VrD.qrD, VrD.rrD]';    % relative acceleration
Tau = [tau.X,tau.Y,tau.Z,tau.K,tau.M,tau.N]';   % thrust forces and moments vector
tauExt = [tauExt.Xe,tauExt.Ye,tauExt.Ze,tauExt.Ke,tauExt.Me,tauExt.Ne]';    % External/tether forces and moments vector
MRB = Mrb(rb);             
CRB = Crb(rb,Vb);
MA = Ma(hyd);
CA = Ca(hyd,Vr);
Dl = DL(hyd);
Dnl = DNL(hyd,Vr);
g_ita = hydStat(ita,rb,phy,hyd);


y = (-(CRB*vb) - MA*vrd - (CA*vr) - ((Dl+Dnl)*vr) - g_ita + Tau + tauExt)./(MRB*ones(6,1));

% Velocity in BODY or {b} frame

VbD.uD = y(1);
VbD.vD = y(2);
VbD.wD = y(3);
VbD.pD = y(4);
VbD.qD = y(5);
VbD.rD = y(6);

== matlab function ROV_Simulation_openloop_ver3_1/Ocean Currents/NED 2 BODY ==
  data: Vcn input Bus: Vcn; ita input Bus: ita; Vcb output Bus: Vcb
function Vcb = e2b(Vcn,ita)

% Rotation matrix 
Rbn = rotbn(ita.phi,ita.theta,ita.psi);
x = [Vcn.ucn;Vcn.vcn;Vcn.wcn];
tmp = Rbn' * x;       

% Velocity of currents in {b} frame
Vcb.uc = tmp(1);
Vcb.vc = tmp(2);
Vcb.wc = tmp(3);
